simulink model "clik_phi_inverse"  (R2022b)
settings: Solver=VariableStepAuto  StartTime=0.0  StopTime=4.0  RelTol=1e-3
undefined symbols (not defined in the file): DiscIntNeverNeededParam, q0, Tc
settings Model: Creator=josh7  LastModifiedBy=brigh
settings SolverCC: AlgebraicLoopSolver=TrustRegion
settings DebuggingCC: UnconnectedInputMsg=warning  UnconnectedOutputMsg=warning  UnconnectedLineMsg=warning  SFMachineParentedDataDiag=warning  ArithmeticOperatorsInVariantConditions=warning
settings ModelReferenceCC: EnableRefExpFcnMdlSchedulingChecks=on
settings SFSimCC: CustomCodeUndefinedFunction=UseInterfaceOnly

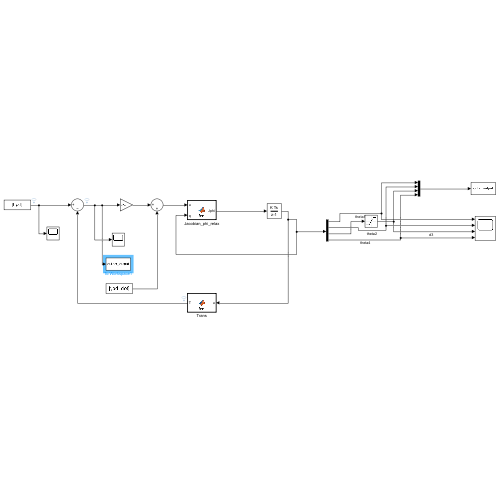
[thumbnail: Simulink's stored preview of the top-level diagram]
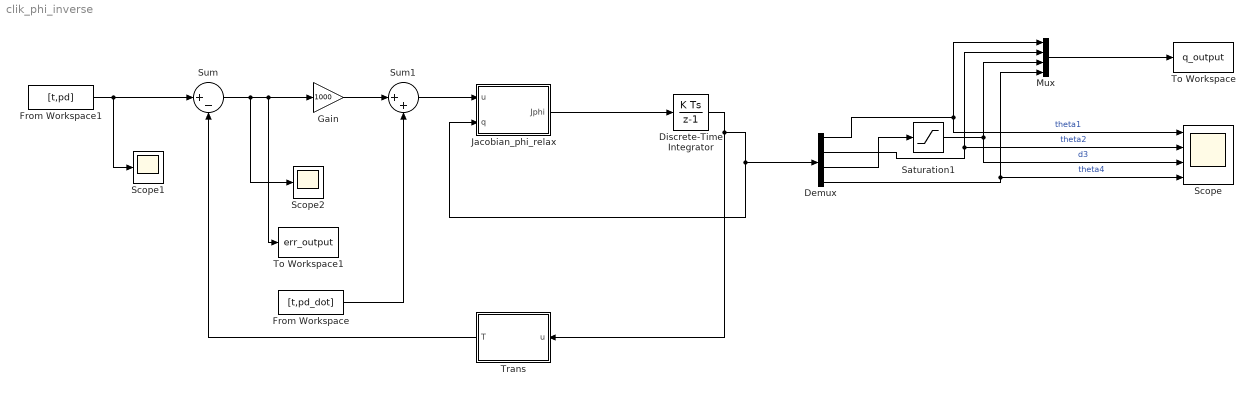
== system clik_phi_inverse ==
  Demux : Demux
  Discrete-Time Integrator : DiscreteIntegrator  InitialCondition=q0  SampleTime=Tc  ICPrevOutput=DiscIntNeverNeededParam  ICPrevScaledInput=DiscIntNeverNeededParam
  From Workspace : FromWorkspace  VariableName=[t,pd_dot]  SampleTime=Tc
  From Workspace1 : FromWorkspace  VariableName=[t,pd]  SampleTime=Tc
  Gain : Gain  Gain=1000
  Jacobian_phi_relax : MATLAB Function  TreatAsAtomicUnit=on
  Mux : Mux
  Saturation1 : Saturate  UpperLimit=1  LowerLimit=0.25
  Scope : Scope  NumInputPorts=4
  Scope1 : Scope
  Scope2 : Scope
  Sum : Sum  Inputs=|+-
  Sum1 : Sum  Inputs=|++
  To Workspace : ToWorkspace  VariableName=q_output  SampleTime=-1
  To Workspace1 : ToWorkspace  VariableName=err_output  SampleTime=-1
  Trans : MATLAB Function  TreatAsAtomicUnit=on
  wires:
  Sum1/1 -> Jacobian_phi_relax/1(u)
  Trans/1(T) -> Sum/2
  Sum/1 -> To Workspace1/1, Gain/1, Scope2/1
  From Workspace1/1 -> Sum/1, Scope1/1
  From Workspace/1 -> Sum1/2
  Gain/1 -> Sum1/1
  Jacobian_phi_relax/1(Jphi) -> Discrete-Time Integrator/1
  Discrete-Time Integrator/1 -> Trans/1(u), Demux/1, Jacobian_phi_relax/2(q)
  Demux/1 -> Mux/1, Scope/1  "theta1"
  Demux/2 -> Mux/2, Scope/2  "theta2"
  Demux/4 -> Mux/4, Scope/4  "theta4"
  Demux/3 -> Saturation1/1
  Saturation1/1 -> Mux/3, Scope/3  "d3"
  Mux/1 -> To Workspace/1

== matlab function clik_phi_inverse/Jacobian_phi_relax ==
  data: u input; Jphi output; q input
function Jphi = fcn(u,q)

a1 = 0.5;
a2 = 0.5;

theta1=q(1);
theta12 = q(1)+q(2);

cos1 = cos(theta1);
sin1 = sin(theta1);

cos12 = cos(theta12);
sin12 = sin(theta12);

K = 10;

J = [-a2*sin12-a1*sin1 -a2*sin12 0 0; a2*cos12+a1*cos1 a2*cos12 0 0; 0 0 1 0];

w = J.';
x = w * inv(J*w);
l = x * u;

c = [1 0 0 0; 0 1 0 0; 0 0 1 0; 0 0 0 1] - (x * J);

q0_dot=K * [(-q(1)/(4*(pi)^2));(-4/(9*(pi)^2))*(q(2)+(pi*8));(0.625-q(3))/2.25;-q(4)/(16*(pi)^2)];

Jphi = l + (c * q0_dot);
end

== matlab function clik_phi_inverse/Trans ==
  data: u input; T output
function T = fcn(u)

a1=0.5;
a2=0.5;

utot= u(1) + u(2);

cos1 = cos(u(1));
sin1 = sin(u(1));
cos12 = cos(utot);
sin12 = sin(utot);

d3=u(3);

T= [a2*cos12+a1*cos1; a2*sin12+a1*sin1; d3];
